simulink library "aplib"  (Simulink 10.0)
settings: Solver=VariableStepAuto  StartTime=0.0  StopTime=10.0  RelTol=1e-3
undefined symbols (not defined in the file): Aail, Aelv, Arud, Bail, Belv, Brud, Cail, CD, Celv, Crud, Dail, Delv, Drud, gamgs, HRW, Sgs, Sloc, uaero0, uprop0, xdot0, xgs, xinco, xloc, ymod1A, ymod1S, ymod2A, ymod2S, yrefA, yrefS
libraries: fdctools x42, navlib1 x8, navlib2 x2, wndlib1 x1, wndlib2 x1
(part 1 of 2)
settings Model: Creator=bhisma  LastModifiedBy=bhisma

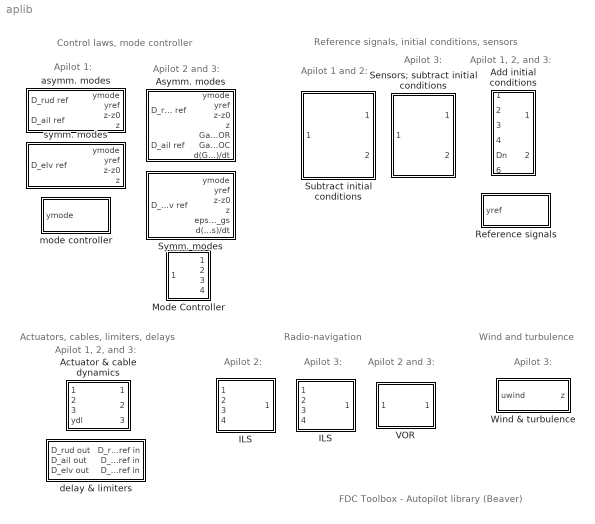
== system aplib ==
  note: Control laws, mode controller
  note: Apilot 1:
  note: Apilot 2 and 3:
  note: Reference signals, initial conditions, sensors
  note: Apilot 1, 2, and 3:
  note: Apilot 1 and 2:
  note: Apilot 3:
  note: Apilot 1, 2, and 3:
  note: Apilot 2:
  note: Radio-navigation
  note: Apilot 2 and 3:
  note: Apilot 3:
  note: FDC Toolbox - Autopilot library (Beaver)
  note: Actuators, cables, limiters, delays
  note: Apilot 3:
  note: Wind and turbulence
  Actuator & cable dynamics : Subsystem  mask(Actuator and cable dynamics){}
      mask help: Dynamics of the actuator/cable system of the Beaver autopilot system.
      mask Help: eval('browse actuatr');
      mask Display: disp('Actuator &\ncable dy-\nnamics')
  Add initial conditions : Subsystem
      mask Display: disp('Add\ninitial\ninputs')
  Asymm. modes : Subsystem  mask(Asymmetrical autopilot modes){}
      mask help:
      | Roll Attitude Hold (RAH) + turn-coordinator
      | Heading Hold/Heading Select (HH)
      | VOR navigation (NAV)
      | Localizer (LOC)
      mask Help: eval('browse ap_asymm')
      mask Display: disp('Asymmetrical\nautopilot\nmodes')
  ILS : Subsystem
      mask Display: plot(0,0,100,100,[53,23,30,61,53],[45,60,64,49,45],[16,27,32,26],[48,40,43,47],[21,20,24,26,21],[44,55,56,47,44],[20,20,16],[50,50,48],[38,27,26,33],[52,46,48,55],[42,38,27],[50,47,46],[40,44,44,45,45,44,42],[48,44,42,42,44,44,50],[47,45,43],[55,58,58],[54,84,98,90,54],[36,21,56,58,36],[74,68],[34,29],[81,76],[43,38],[87,83],[49,45],[94,89],[57,52],[105,105],[0,0])
  "ILS " : Subsystem
      mask Display: plot(0,0,100,100,[53,23,30,61,53],[45,60,64,49,45],[16,27,32,26],[48,40,43,47],[21,20,24,26,21],[44,55,56,47,44],[20,20,16],[50,50,48],[38,27,26,33],[52,46,48,55],[42,38,27],[50,47,46],[40,44,44,45,45,44,42],[48,44,42,42,44,44,50],[47,45,43],[55,58,58],[54,84,98,90,54],[36,21,56,58,36],[74,68],[34,29],[81,76],[43,38],[87,83],[49,45],[94,89],[57,52],[105,105],[0,0])
  Mode Controller : Subsystem  mask(Mode Controller){}
      mask help: Mode Controller, allows VOR navigation, Localizer, and Glideslope modes to switch from 'Armed' to 'Coupled'.
      mask Help: eval('browse modectrl')
      mask Display: disp('Mode\nCon-\ntroller')
  Reference signals : Subsystem  mask(Reference signals){}
      mask help: Reference signals for Beaver autopilot
      mask Help: eval('browse refsgnls.htm')
      mask Display: disp('Reference\nsignals')
  Sensors; subtract initial conditions : Subsystem
      mask Display: disp('Sensors\n\nsubtract\ninitial\nconditions')
  Subtract initial conditions : Subsystem
      mask Display: disp('Subtract\ninitial con-\nditions\n\nNo sensors!')
  Symm. modes : Subsystem  mask(Symmetrical autopilot modes){}
      mask help:
      | Pitch Attitude Hold (PAH) + turn-compensator
      | Altitude Hold (ALH)
      | Altitude Select (ALS)
      | Glideslope (GS)
      mask Help: eval('browse ap_symm')
      mask Display: disp('Symmetrical\nautopilot\nmodes')
  VOR : Subsystem
      mask Display: plot(0,0,100,100,[86,85,90,86,80,85,0],[16,80,20,16,20,80,62],[22,18,25,28,22,19],[36,32,29,33,36,45],[17,15,12,18,16,19],[37,37,34,32,44,46],[22,31,47,52,19,15,28,22],[36,44,39,44,55,50,45,38],[31,28],[44,45],[20,18,17],[31,30,32],[36,35,36,37,36,35,35,35,33,31,25],[41,38,33,32,30,30,32,33,37,35,34],[85,42],[80,50],[86,87,87,86,84,83,84,85],[83,81,78,76,76,79,82,83])
  Wind & turbulence : Subsystem
      mask Display: disp('Wind &\nturbulence')
  asymm. modes : Subsystem  mask(Asymmetrical autopilot modes){}
      mask help:
      | Roll Attitude Hold (RAH) + turn-coordinator
      | Heading Hold/Heading Select (HH)
      mask Help: eval('browse ap_asymm')
      mask Display: disp('Asymmetrical\nautopilot modes')
  delay & limiters : Subsystem  mask(Computational delay and limiters){}
      mask help: Computational delay and hardware-related limiters for the Beaver autopilot system.
      mask Help: eval('browse delaylim')
      mask Display: disp('Computational\ndelay & limiters')
  mode controller : Subsystem  mask(Mode Controller){}
      mask help: 'Dummy' Mode Controller (no mode-switching).
      mask Help: eval('browse modectrl')
      mask Display: disp('Mode\nController')
  symm. modes : Subsystem  mask(Symmetrical autopilot modes){}
      mask help:
      | Pitch Attitude Hold (PAH) + turn-compensator
      | Altitude Hold (ALH)
      | Altitude Select (ALS)
      mask Help: eval('browse ap_symm')
      mask Display: disp('Symmetrical\nautopilot modes')

== system aplib/Actuator & cable dynamics ==
  VDdeltae : Inport
  VDdeltaa : Inport  Port=2
  VDdeltar : Inport  Port=3
  ydl : Inport  Port=4
  Ailerons actuator and cables : StateSpace  A=Aail  B=Bail  C=Cail  D=Dail  InitialCondition=0
  Demux1 : Demux  Outputs=3
  Elevator actuator and cables : StateSpace  A=Aelv  B=Belv  C=Celv  D=Delv  InitialCondition=0
  Mux : Mux  Inputs=2
  Mux4 : Mux  Inputs=2
  Mux5 : Mux  Inputs=2
  Rudder actuator and cables : StateSpace  A=Arud  B=Brud  C=Crud  D=Drud  InitialCondition=0
  t1 : Subsystem
      settings: OpenFcn=browse actuatr
      mask Display: disp('Dynamics of the actuators and cables\nfor elevator, ailerons, and rudder.\nM.O. Rauw, January 2004')
  Ddeltae : Outport
  Ddeltaa : Outport  Port=2
  Ddeltar : Outport  Port=3
  wires:
  VDdeltae/1 -> Mux5/1
  VDdeltaa/1 -> Mux/1
  VDdeltar/1 -> Mux4/1
  Ailerons actuator and cables/1 -> Ddeltaa/1
  Rudder actuator and cables/1 -> Ddeltar/1
  Elevator actuator and cables/1 -> Ddeltae/1
  ydl/1 -> Demux1/1
  Demux1/3 -> Mux4/2  "rb/2V"
  Demux1/1 -> Mux/2  "pb/2V"
  Demux1/2 -> Mux5/2  "qc/V"
  Mux/1 -> Ailerons actuator and cables/1
  Mux4/1 -> Rudder actuator and cables/1
  Mux5/1 -> Elevator actuator and cables/1

== system aplib/Add initial conditions ==
  note: Add initial inputs
  note: ENGINE INPUTS:
  note: AERODYNAMIC INPUTS:
  Ddeltae : Inport
  Ddeltaa : Inport  Port=2
  Ddeltar : Inport  Port=3
  Ddeltaf : Inport  Port=4
  Dn : Inport  Port=5
  Dpz : Inport  Port=6
  Initial inputs for aeromod : Constant  Value=uaero0
  Initial inputs for engmod : Constant  Value=uprop0
  Mux1 : Mux
  Mux2 : Mux  Inputs=2
  Sum : Sum  SaturateOnIntegerOverflow=on  InputSameDT=on  OutDataTypeStr=Inherit: Same as first input
  Sum1 : Sum  SaturateOnIntegerOverflow=on  InputSameDT=on  OutDataTypeStr=Inherit: Same as first input
  uaero : Outport
  uprop : Outport  Port=2
  wires:
  Ddeltaa/1 -> Mux1/2
  Ddeltae/1 -> Mux1/1
  Ddeltar/1 -> Mux1/3
  Ddeltaf/1 -> Mux1/4
  Initial inputs for engmod/1 -> Sum/2
  Mux2/1 -> Sum/1
  Dpz/1 -> Mux2/2
  Dn/1 -> Mux2/1
  Initial inputs for aeromod/1 -> Sum1/1
  Sum1/1 -> uaero/1
  Mux1/1 -> Sum1/2
  Sum/1 -> uprop/1

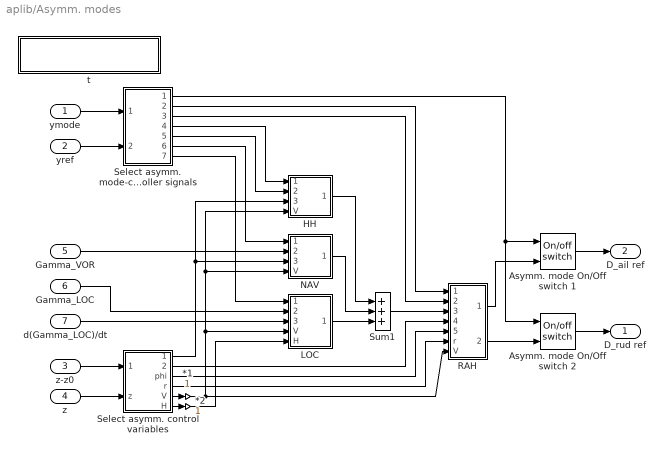
== system aplib/Asymm. modes ==
  ymode : Inport
  yref : Inport  Port=2
  z-z0 : Inport  Port=3
  z : Inport  Port=4
  Gamma_VOR : Inport  Port=5
  Gamma_LOC : Inport  Port=6
  d(Gamma_LOC)/dt : Inport  Port=7
  *1 : Gain  SaturateOnIntegerOverflow=on  OutDataTypeStr=Inherit: Same as input  ParamDataTypeStr=Inherit: Same as input
  *2 : Gain  SaturateOnIntegerOverflow=on  OutDataTypeStr=Inherit: Same as input  ParamDataTypeStr=Inherit: Same as input
  "Asymm. mode On/Off switch 1 " : fdctools/On//off switch
  Asymm. mode On/Off switch 2 : fdctools/On//off switch
  HH : Subsystem
  LOC : Subsystem
  NAV : Subsystem
  RAH : Subsystem
  Select asymm. control variables : Subsystem
  Select asymm. mode-controller signals : Subsystem
  Sum1 : Sum  Inputs=+++  SaturateOnIntegerOverflow=on  InputSameDT=on  OutDataTypeStr=Inherit: Same as first input
  t : Subsystem
      settings: OpenFcn=browse ap_asymm
      mask Display: disp('Asymm. autopilot modes\nMarc Rauw, March 2004')
  D_rud ref : Outport
  D_ail ref : Outport  Port=2
  wires:
  d(Gamma_LOC)/dt/1 -> LOC/3(d(Gamma_loc)/dt)
  Gamma_LOC/1 -> LOC/2(Gamma_loc)
  Gamma_VOR/1 -> NAV/2(Gamma_VOR)
  Select asymm. mode-controller signals/5(Dpsir (HH)) -> HH/2(Dpsir (HH))
  Sum1/1 -> RAH/3(Dphir (outer loop))
  *2/1 -> LOC/5(H)
  *1/1 -> RAH/7(V), LOC/4(V), HH/4(V), NAV/4(V)
  Select asymm. control variables/6(H) -> *2/1
  Select asymm. mode-controller signals/7(LOC coupled?) -> LOC/1(LOC coupled?)
  Select asymm. mode-controller signals/6(NAV?) -> NAV/1(NAV?)
  Select asymm. mode-controller signals/4(HH?) -> HH/1(HH?)
  Select asymm. mode-controller signals/3(Dphir (RAH)) -> RAH/2(Dphir (RAH))
  Select asymm. mode-controller signals/2(Asymm. outer loop?) -> RAH/1(Asymm.  outer loop?)
  Select asymm. control variables/2(phi-phi0) -> RAH/4(phi-phi0)
  Select asymm. control variables/3(phi) -> RAH/5(phi)
  Select asymm. control variables/4(r) -> RAH/6(r)
  Select asymm. control variables/5(V) -> *1/1
  LOC/1(Dphir (LOC)) -> Sum1/3
  NAV/1(Dphir (NAV)) -> Sum1/2
  Select asymm. control variables/1(psi-psi0) -> HH/3(psi-psi0), NAV/3(psi-psi0)
  RAH/1(D_ail ref) -> "Asymm. mode On/Off switch 1 "/2
  RAH/2(D_rud ref) -> Asymm. mode On/Off switch 2/2
  HH/1(Dphir (HH)) -> Sum1/1
  Select asymm. mode-controller signals/1(Asymm. mode?) -> "Asymm. mode On/Off switch 1 "/1, Asymm. mode On/Off switch 2/1
  ymode/1 -> Select asymm. mode-controller signals/1(ymode)
  yref/1 -> Select asymm. mode-controller signals/2(yref)
  Asymm. mode On/Off switch 2/1 -> D_rud ref/1
  "Asymm. mode On/Off switch 1 "/1 -> D_ail ref/1
  z/1 -> Select asymm. control variables/2(z)
  z-z0/1 -> Select asymm. control variables/1(z-z0)

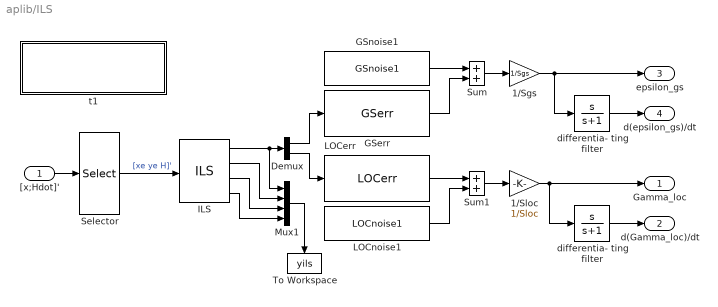
== system aplib/ILS ==
  "[x;Hdot]'" : Inport
  1/Sgs : Gain  Gain=1/Sgs  SaturateOnIntegerOverflow=on  OutDataTypeStr=Inherit: Same as input  ParamDataTypeStr=Inherit: Same as input
  1/Sloc : Gain  Gain=1/Sloc  SaturateOnIntegerOverflow=on  OutDataTypeStr=Inherit: Same as input  ParamDataTypeStr=Inherit: Same as input
  Demux : Demux  Outputs=2
  GSerr : navlib1/GSerr  cat=2  MaskParam2=0  MaskParam3=0  MaskParam4=-3
  GSnoise1 : navlib1/GSnoise1  Lgs=85  sigma_gs=15  V=30
  ILS : navlib1/ILS  RWpos=[12000,0,0]  MaskParam1=0  MaskParam3=3000  MaskParam4=300  MaskParam5=-100  MaskParam6=-3
  LOCerr : navlib1/LOCerr  cat=2  xloc=3000  MaskParam2=0  MaskParam3=0
  LOCnoise1 : navlib1/LOCnoise1  Lloc=130  sigma_loc=15  V=30
  Mux1 : Mux  Inputs=[2 2 6 2]
  Selector : Selector  InputPortWidth=13  IndexOptions=Index vector (dialog)  Indices=[10 11 12]  OutputSizes=1
  Sum : Sum  SaturateOnIntegerOverflow=on  InputSameDT=on  OutDataTypeStr=Inherit: Same as first input
  Sum1 : Sum  SaturateOnIntegerOverflow=on  InputSameDT=on  OutDataTypeStr=Inherit: Same as first input
  To Workspace : ToWorkspace  VariableName=yils
      settings: MaxDataPoints=5000
  differentia- ting filter : TransferFcn  Numerator=[1 0]  Denominator=[1 1]
  "differentia- ting filter " : TransferFcn  Numerator=[1 0]  Denominator=[1 1]
  t1 : Subsystem
      settings: OpenFcn=browse ilsxmpl
      mask Display: disp('ILS signals for autopilot\n(with noise!)\nMarc Rauw, April 2004')
  Gamma_loc : Outport
  d(Gamma_loc)/dt : Outport  Port=2
  epsilon_gs : Outport  Port=3
  d(epsilon_gs)/dt : Outport  Port=4
  wires:
  Selector/1 -> ILS/1  "[xe ye H]'"
  Demux/2 -> LOCerr/1
  Demux/1 -> GSerr/1
  Mux1/1 -> To Workspace/1
  GSnoise1/1 -> Sum/1
  GSerr/1 -> Sum/2
  Sum/1 -> 1/Sgs/1
  1/Sgs/1 -> epsilon_gs/1, differentia- ting filter/1
  differentia- ting filter/1 -> d(epsilon_gs)/dt/1
  LOCerr/1 -> Sum1/1
  LOCnoise1/1 -> Sum1/2
  1/Sloc/1 -> Gamma_loc/1, "differentia- ting filter "/1
  "differentia- ting filter "/1 -> d(Gamma_loc)/dt/1
  Sum1/1 -> 1/Sloc/1
  ILS/2 -> Mux1/2
  ILS/3 -> Mux1/3
  ILS/1 -> Mux1/1, Demux/1
  ILS/4 -> Mux1/4
  "[x;Hdot]'"/1 -> Selector/1

== system aplib/ILS  ==
  "[x;Hdot]'" : Inport
  1/Sgs : Gain  Gain=1/Sgs  SaturateOnIntegerOverflow=on  OutDataTypeStr=Inherit: Same as input  ParamDataTypeStr=Inherit: Same as input
  1/Sloc : Gain  Gain=1/Sloc  SaturateOnIntegerOverflow=on  OutDataTypeStr=Inherit: Same as input  ParamDataTypeStr=Inherit: Same as input
  Demux : Demux  Outputs=2
  GSerr : navlib1/GSerr  cat=2  MaskParam2=0  MaskParam3=0  MaskParam4=-3
  ILS : navlib1/ILS  RWpos=[12000,0,0]  MaskParam1=0  MaskParam3=3000  MaskParam4=300  MaskParam5=-100  MaskParam6=-3
  LOCerr : navlib1/LOCerr  cat=2  xloc=3000  MaskParam2=0  MaskParam3=0
  Mux1 : Mux  Inputs=[2 2 6 2]
  Selector : Selector  InputPortWidth=13  IndexOptions=Index vector (dialog)  Indices=[10 11 12]  OutputSizes=1
  To Workspace : ToWorkspace  VariableName=yils
      settings: MaxDataPoints=5000
  differentia- ting filter : TransferFcn  Numerator=[1 0]  Denominator=[1 1]
  "differentia- ting filter " : TransferFcn  Numerator=[1 0]  Denominator=[1 1]
  t1 : Subsystem
      settings: OpenFcn=browse ilsxmpl
      mask Display: disp('ILS signals for autopilot\n(no noise!)\nMarc Rauw, May 2004')
  Gamma_loc : Outport
  d(Gamma_loc)/dt : Outport  Port=2
  epsilon_gs : Outport  Port=3
  d(epsilon_gs)/dt : Outport  Port=4
  wires:
  "[x;Hdot]'"/1 -> Selector/1
  Selector/1 -> ILS/1  "[xe ye H]'"
  Mux1/1 -> To Workspace/1
  Demux/1 -> GSerr/1
  Demux/2 -> LOCerr/1
  ILS/4 -> Mux1/4
  ILS/1 -> Demux/1, Mux1/1
  ILS/3 -> Mux1/3
  ILS/2 -> Mux1/2
  GSerr/1 -> 1/Sgs/1
  1/Sgs/1 -> epsilon_gs/1, differentia- ting filter/1
  LOCerr/1 -> 1/Sloc/1
  1/Sloc/1 -> Gamma_loc/1, "differentia- ting filter "/1
  "differentia- ting filter "/1 -> d(Gamma_loc)/dt/1
  differentia- ting filter/1 -> d(epsilon_gs)/dt/1

== system aplib/Mode Controller ==
  Gamma_VOR : Inport
  d(Gamma_loc)/dt : Inport  Port=2
  Gamma_loc : Inport  Port=3
  epsilon_gs : Inport  Port=4
  Asymmetrical mode switch : Subsystem
      mask Display: disp('Armed->Coupled\nswitch for\nasymmetrical mode(s)')
  Asymmetrical mode switch1 : Subsystem
      mask Display: disp('Armed->Coupled\nswitch for\nsymmetrical mode(s)')
  GS mode active? : Constant  Value=ymod2S(5)
  GS mode status : Subsystem
      mask Display: disp('Glideslope\nmode status')
  LOC mode active? : Constant  Value=ymod2A(5)
  LOC mode status : Subsystem
      mask Display: disp('Localizer\nmode status')
  Mux1 : Mux  Inputs=[5 5]
  NAV mode active? : Constant  Value=ymod2A(4)
  NAV mode status : Subsystem
      mask Display: disp('VOR-navigation\nmode status')
  Sum : Sum  SaturateOnIntegerOverflow=on  InputSameDT=on  OutDataTypeStr=Inherit: Same as first input
  t : Subsystem
      settings: OpenFcn=browse modectrl
      mask Display: disp('Mode-controller\nM.O. Rauw, April 2004')
  ymode : Outport
  wires:
  Mux1/1 -> ymode/1
  Asymmetrical mode switch/1(ymode_asymm) -> Mux1/2
  Asymmetrical mode switch1/1(ymode_symm) -> Mux1/1
  GS mode status/1(GS status) -> Asymmetrical mode switch1/1(Symmetrical mode-status)
  epsilon_gs/1 -> GS mode status/1(epsilon_gs)
  GS mode active?/1 -> GS mode status/Enable
  Sum/1 -> Asymmetrical mode switch/1(Asymmetrical mode status)
  LOC mode status/1(LOC status) -> Sum/2
  Gamma_VOR/1 -> NAV mode status/1(Gamma_VOR)
  NAV mode active?/1 -> NAV mode status/Enable
  d(Gamma_loc)/dt/1 -> LOC mode status/2(d(Gamma_loc)/dt)
  Gamma_loc/1 -> LOC mode status/1(Gamma_loc)
  LOC mode active?/1 -> LOC mode status/Enable
  NAV mode status/1(NAV status) -> Sum/1

== system aplib/Reference signals ==
  Constant : Constant  Value=[yrefS;yrefA]
  t : Subsystem
      settings: OpenFcn=browse modectrl
      mask Display: disp('Reference signals\nMarc Rauw, April 2004')
  yref : Outport
  wires:
  Constant/1 -> yref/1

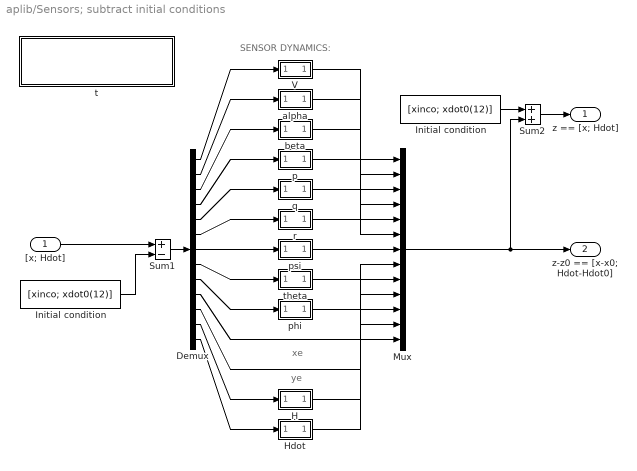
== system aplib/Sensors; subtract initial conditions ==
  note: SENSOR DYNAMICS:
  note: xe
  note: ye
  "[x; Hdot]" : Inport
  Demux : Demux  Outputs=13
  H : Subsystem
  Hdot : Subsystem
  Initial condition : Constant  Value=[xinco; xdot0(12)]
  "Initial condition " : Constant  Value=[xinco; xdot0(12)]
  Mux : Mux  Inputs=13
  Sum1 : Sum  Inputs=+-  SaturateOnIntegerOverflow=on  InputSameDT=on  OutDataTypeStr=Inherit: Same as first input
  Sum2 : Sum  SaturateOnIntegerOverflow=on  InputSameDT=on  OutDataTypeStr=Inherit: Same as first input
  V : Subsystem
  alpha : Subsystem
  beta : Subsystem
  p : Subsystem
  phi : Subsystem
  psi : Subsystem
  q : Subsystem
  r : Subsystem
  t : Subsystem
      settings: OpenFcn=browse sensors
      mask Display: disp('Include sensormodels\nhere (no VOR/ILS)!\nMarc Rauw, February 2004')
  theta : Subsystem
  "z == [x; Hdot] " : Outport
  z-z0 == [x-x0; Hdot-Hdot0] : Outport  Port=2
  wires:
  Sum1/1 -> Demux/1
  "[x; Hdot]"/1 -> Sum1/1
  Initial condition/1 -> Sum1/2
  Hdot/1(Hdot out) -> Mux/13
  H/1(H out) -> Mux/12
  V/1(V out) -> Mux/1
  alpha/1(alpha out) -> Mux/2
  beta/1(beta out) -> Mux/3
  p/1(p out) -> Mux/4
  q/1(q out) -> Mux/5
  r/1(r out) -> Mux/6
  psi/1(psi out) -> Mux/7
  theta/1(theta out) -> Mux/8
  phi/1(phi out) -> Mux/9
  Demux/13 -> Hdot/1(Hdot in)
  Demux/12 -> H/1(H in)
  Demux/11 -> Mux/11
  Demux/10 -> Mux/10
  Demux/9 -> phi/1(phi in)
  Demux/8 -> theta/1(theta in)
  Demux/7 -> psi/1(psi in)
  Demux/6 -> r/1(r in)
  Demux/5 -> q/1(q in)
  Demux/4 -> p/1(p in)
  Demux/3 -> beta/1(beta in)
  Demux/2 -> alpha/1(alpha in)
  Demux/1 -> V/1(V in)
  "Initial condition "/1 -> Sum2/1
  Sum2/1 -> "z == [x; Hdot] "/1
  Mux/1 -> Sum2/2, z-z0 == [x-x0; Hdot-Hdot0]/1

== system aplib/Subtract initial conditions ==
  note: Subtract initial conditions
  "[x; Hdot]" : Inport
  Initial condition : Constant  Value=[xinco; xdot0(12)]
  Sum : Sum  Inputs=+-  SaturateOnIntegerOverflow=on  InputSameDT=on  OutDataTypeStr=Inherit: Same as first input
  "z == [x; Hdot] " : Outport
  z-z0 == [x-x0; Hdot-Hdot0] : Outport  Port=2
  wires:
  "[x; Hdot]"/1 -> "z == [x; Hdot] "/1, Sum/1
  Initial condition/1 -> Sum/2
  Sum/1 -> z-z0 == [x-x0; Hdot-Hdot0]/1

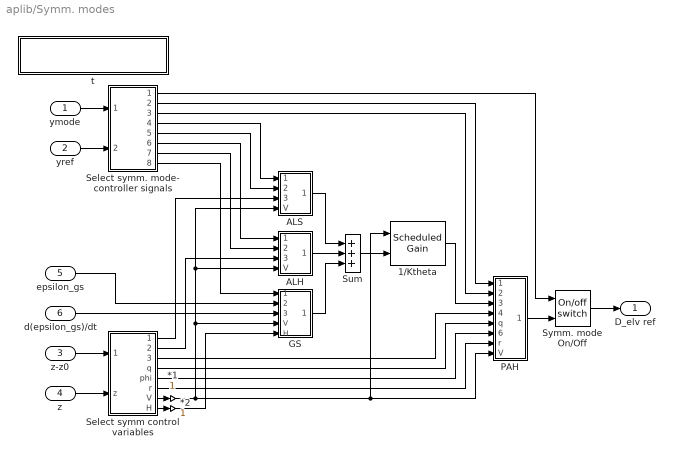
== system aplib/Symm. modes ==
  ymode : Inport
  yref : Inport  Port=2
  z-z0 : Inport  Port=3
  z : Inport  Port=4
  epsilon_gs : Inport  Port=5
  d(epsilon_gs)/dt : Inport  Port=6
  *1 : Gain  SaturateOnIntegerOverflow=on  OutDataTypeStr=Inherit: Same as input  ParamDataTypeStr=Inherit: Same as input
  *2 : Gain  SaturateOnIntegerOverflow=on  OutDataTypeStr=Inherit: Same as input  ParamDataTypeStr=Inherit: Same as input
  1/Ktheta : fdctools/Scheduled Gain  K=1/(-1.375*10^(-3)*u[1]^2 + 0.1575*u[1] - 4.8031)
  ALH : Subsystem
  ALS : Subsystem
  GS : Subsystem
  PAH : Subsystem
  Select symm control variables : Subsystem
  Select symm. mode- controller signals : Subsystem
  Sum : Sum  Inputs=+++  SaturateOnIntegerOverflow=on  InputSameDT=on  OutDataTypeStr=Inherit: Same as first input
  Symm. mode On/Off : fdctools/On//off switch
  t : Subsystem
      settings: OpenFcn=browse ap_symm
      mask Display: disp('Symm. autopilot modes\nMarc Rauw, March 2004')
  D_elv ref : Outport
  wires:
  epsilon_gs/1 -> GS/2(epsilon_gs)
  d(epsilon_gs)/dt/1 -> GS/3(d(epsilon_gs)/dt)
  *1/1 -> ALS/4(V), ALH/4(V), GS/4(V), PAH/8(V), 1/Ktheta/1
  1/Ktheta/1 -> PAH/3(Dthetar (outer loop))
  GS/1(Dthetar (GS)) -> Sum/3
  ALS/1(Dthetar (ALS)) -> Sum/1
  ALH/1(Dthetar (ALH)) -> Sum/2
  Select symm control variables/1(Hdot-Hdot0) -> ALS/3(Hdot-Hdot0)
  Select symm control variables/2(H-H0) -> ALH/3(H-H0)
  Select symm control variables/3(theta-theta0) -> PAH/4(theta-theta0)
  Select symm control variables/4(q) -> PAH/5(q)
  Select symm control variables/5(phi) -> PAH/6(phi)
  Select symm control variables/6(r) -> PAH/7(r)
  Select symm control variables/7(V) -> *1/1
  Select symm. mode- controller signals/2(Symm. outer loop?) -> PAH/1(Symm.  outer loop?)
  Select symm. mode- controller signals/3(Dthetar (PAH)) -> PAH/2(Dthetar (PAH/GA))
  Select symm. mode- controller signals/4(ALS?) -> ALS/1(ALS?)
  Select symm. mode- controller signals/5(DHdot r (ALS)) -> ALS/2(DHdot r (ALS))
  Select symm. mode- controller signals/6(ALH?) -> ALH/1(ALH?)
  Select symm. mode- controller signals/7(DHr (ALH)) -> ALH/2(DHr (ALH))
  Select symm control variables/8(H) -> *2/1
  *2/1 -> GS/5(H)
  Select symm. mode- controller signals/8(GS coupled?) -> GS/1(GS coupled?)
  Select symm. mode- controller signals/1(Symm. mode?) -> Symm. mode On/Off/1
  PAH/1(D_elv ref) -> Symm. mode On/Off/2
  Symm. mode On/Off/1 -> D_elv ref/1
  yref/1 -> Select symm. mode- controller signals/2(yref)
  ymode/1 -> Select symm. mode- controller signals/1(ymode)
  z-z0/1 -> Select symm control variables/1(z-z0)
  z/1 -> Select symm control variables/2(z)
  Sum/1 -> 1/Ktheta/2

== system aplib/VOR ==
  "[x' ; Hdot]'" : Inport
  Demux : Demux  Outputs=[3 1]
  Mux1 : Mux  Inputs=[1 1 2 1]
  Selector : Selector  InputPortWidth=13  IndexOptions=Index vector (dialog)  Indices=[10 11 12 7]  OutputSizes=1
  To Workspace : ToWorkspace  VariableName=yvor
      settings: MaxDataPoints=5000
  VOR : navlib2/VOR  xVOR=xVOR  yVOR=yVOR  HVOR=HVOR  CD=CD
  VORerr : navlib2/VORerr  MaskParam1=0
  t : Subsystem
      settings: OpenFcn=browse vorxmpl
      mask Display: disp('VOR signals\nMarc Rauw, February 2004')
  Gamma_VOR : Outport
  wires:
  "[x' ; Hdot]'"/1 -> Selector/1
  Selector/1 -> Demux/1
  Demux/1 -> VOR/1  "[xe ye H]'"
  Demux/2 -> VOR/2  "psi"
  VORerr/1 -> Mux1/1, Gamma_VOR/1
  VOR/4 -> Mux1/4
  VOR/3 -> Mux1/3
  VOR/2 -> Mux1/2
  Mux1/1 -> To Workspace/1
  VOR/1 -> VORerr/1

== system aplib/Wind & turbulence ==
  z : Inport
  BLwind : wndlib1/BLwind  Vw=1*(u[1]^0.2545 - 0.4097)/1.3470  psi_w=180  theta_w=0
  Demux : Demux  Outputs=[12 1]
  Demux1 : Demux  Outputs=[1 11]
  Mux1 : Mux  Inputs=[3 3]
  Sum : Sum  SaturateOnIntegerOverflow=on  InputSameDT=on  OutDataTypeStr=Inherit: Same as first input
  Terminator_1 : Terminator
  Terminator_2 : Terminator
  deriv : Derivative
  t : Subsystem
      mask Display: disp('Wind and turbulence\nMarc Rauw, April 2003')
  turb2 : wndlib2/turb2
  uwind : Outport
  wires:
  BLwind/1 -> deriv/1, Mux1/1
  deriv/1 -> Mux1/2
  Sum/1 -> uwind/1
  turb2/1 -> Sum/1
  Mux1/1 -> Sum/2
  Demux1/1 -> turb2/1  "V"
  Demux1/2 -> Terminator_2/1
  z/1 -> Demux/1
  Demux/1 -> Demux1/1, BLwind/1  "x"
  Demux/2 -> Terminator_1/1

== system aplib/asymm. modes ==
  ymode : Inport
  yref : Inport  Port=2
  z-z0 : Inport  Port=3
  z : Inport  Port=4
  *1 : Gain  SaturateOnIntegerOverflow=on  OutDataTypeStr=Inherit: Same as input  ParamDataTypeStr=Inherit: Same as input
  "Asymm. mode On/Off switch 1 " : fdctools/On//off switch
  Asymm. mode On/Off switch 2 : fdctools/On//off switch
  HH : Subsystem
  RAH : Subsystem
  Select asymm. control variables : Subsystem
  Select asymm. mode-controller signals : Subsystem
  Terminator_1 : Terminator
  Terminator_2 : Terminator
  Terminator_3 : Terminator
  t : Subsystem
      settings: OpenFcn=browse ap_asymm
      mask Display: disp('Asymm. autopilot modes\n(without NAV and LOC modes)\nMarc Rauw, April 2003')
  D_rud ref : Outport
  D_ail ref : Outport  Port=2
  wires:
  *1/1 -> RAH/7(V), HH/4(V)
  RAH/2(D_rud ref) -> Asymm. mode On/Off switch 2/2
  Select asymm. control variables/5(V) -> *1/1
  Select asymm. control variables/4(r) -> RAH/6(r)
  z/1 -> Select asymm. control variables/2(z)
  HH/1(Dphir (HH)) -> RAH/3(Dphir (outer loop))
  Select asymm. control variables/1(psi-psi0) -> HH/3(psi-psi0)
  RAH/1(D_ail ref) -> "Asymm. mode On/Off switch 1 "/2
  Select asymm. control variables/6(H) -> Terminator_1/1
  Asymm. mode On/Off switch 2/1 -> D_rud ref/1
  "Asymm. mode On/Off switch 1 "/1 -> D_ail ref/1
  z-z0/1 -> Select asymm. control variables/1(z-z0)
  Select asymm. control variables/2(phi-phi0) -> RAH/4(phi-phi0)
  Select asymm. control variables/3(phi) -> RAH/5(phi)
  Select asymm. mode-controller signals/2(Asymm. outer loop?) -> RAH/1(Asymm.  outer loop?)
  yref/1 -> Select asymm. mode-controller signals/2(yref)
  ymode/1 -> Select asymm. mode-controller signals/1(ymode)
  Select asymm. mode-controller signals/1(Asymm. mode?) -> Asymm. mode On/Off switch 2/1, "Asymm. mode On/Off switch 1 "/1
  Select asymm. mode-controller signals/3(Dphir (RAH)) -> RAH/2(Dphir (RAH))
  Select asymm. mode-controller signals/4(HH?) -> HH/1(HH?)
  Select asymm. mode-controller signals/5(Dpsir (HH)) -> HH/2(Dpsir (HH))
  Select asymm. mode-controller signals/6(NAV?) -> Terminator_2/1
  Select asymm. mode-controller signals/7(LOC coupled?) -> Terminator_3/1

== system aplib/delay & limiters ==
  D_rud ref in : Inport
  D_ail ref in : Inport  Port=2
  D_elv ref in : Inport  Port=3
  " +/- 10 V " : Saturate  UpperLimit=10 * (pi/180)  LowerLimit=-10 * (pi/180)
  " delay" : TransportDelay  DelayTime=0.03
  +/- 10 V : Saturate  UpperLimit=10 * (pi/180)  LowerLimit=-10 * (pi/180)
  "+/- 10 V " : Saturate  UpperLimit=10 * (pi/180)  LowerLimit=-10 * (pi/180)
  delay : TransportDelay  DelayTime=0.03
  "delay " : TransportDelay  DelayTime=0.03
  t : Subsystem
      settings: OpenFcn=browse delaylim
      mask Display: disp('Computational delay and\ninput limiters (+- 10 Volt)\nMarc Rauw, April 2003')
  D_rud out : Outport
  D_ail out : Outport  Port=2
  D_elv out : Outport  Port=3
  wires:
  D_rud ref in/1 -> delay/1
  delay/1 -> +/- 10 V/1
  D_elv ref in/1 -> " delay"/1
  " +/- 10 V "/1 -> D_elv out/1
  D_ail ref in/1 -> "delay "/1
  "+/- 10 V "/1 -> D_ail out/1
  +/- 10 V/1 -> D_rud out/1
  " delay"/1 -> " +/- 10 V "/1
  "delay "/1 -> "+/- 10 V "/1

== system aplib/mode controller ==
  Mux1 : Mux  Inputs=[5 5]
  asymm. mode-switches : Constant  Value=ymod1A
  symm. mode-switches : Constant  Value=ymod1S
  t : Subsystem
      settings: OpenFcn=browse modectrl
      mask Display: disp('Mode Controller (Mode Select)\nNo on-line mode-switching!\nMarc Rauw, April 2003')
  ymode : Outport
  wires:
  Mux1/1 -> ymode/1
  symm. mode-switches/1 -> Mux1/1
  asymm. mode-switches/1 -> Mux1/2

== system aplib/symm. modes ==
  ymode : Inport
  yref : Inport  Port=2
  z-z0 : Inport  Port=3
  z : Inport  Port=4
  *1 : Gain  SaturateOnIntegerOverflow=on  OutDataTypeStr=Inherit: Same as input  ParamDataTypeStr=Inherit: Same as input
  1/Ktheta : fdctools/Scheduled Gain  K=1/(-1.375*10^(-3)*u[1]^2 + 0.1575*u[1] - 4.8031)
  ALH : Subsystem
  ALS : Subsystem
  PAH : Subsystem
  Select symm control variables : Subsystem
  Select symm. mode- controller signals : Subsystem
  Sum : Sum  SaturateOnIntegerOverflow=on  InputSameDT=on  OutDataTypeStr=Inherit: Same as first input
  Symm. mode On/Off : fdctools/On//off switch
  Terminator_1 : Terminator
  Terminator_2 : Terminator
  t : Subsystem
      settings: OpenFcn=browse ap_symm
      mask Display: disp('Symm. autopilot modes\n(without glideslope mode)\nMarc Rauw, April 2003')
  D_elv ref : Outport
  wires:
  Symm. mode On/Off/1 -> D_elv ref/1
  PAH/1(D_elv ref) -> Symm. mode On/Off/2
  ALH/1(Dthetar (ALH)) -> Sum/2
  Select symm control variables/2(H-H0) -> ALH/3(H-H0)
  Select symm control variables/3(theta-theta0) -> PAH/4(theta-theta0)
  Select symm control variables/4(q) -> PAH/5(q)
  Select symm control variables/5(phi) -> PAH/6(phi)
  Select symm control variables/6(r) -> PAH/7(r)
  Select symm control variables/7(V) -> *1/1
  Select symm. mode- controller signals/4(ALS?) -> ALS/1(ALS?)
  Select symm. mode- controller signals/5(DHdot r (ALS)) -> ALS/2(DHdot r (ALS))
  Select symm. mode- controller signals/6(ALH?) -> ALH/1(ALH?)
  Select symm. mode- controller signals/7(DHr (ALH)) -> ALH/2(DHr (ALH))
  Select symm. mode- controller signals/3(Dthetar (PAH)) -> PAH/2(Dthetar (PAH/GA))
  Select symm. mode- controller signals/2(Symm. outer loop?) -> PAH/1(Symm.  outer loop?)
  Select symm. mode- controller signals/1(Symm. mode?) -> Symm. mode On/Off/1
  Select symm control variables/1(Hdot-Hdot0) -> ALS/3(Hdot-Hdot0)
  *1/1 -> ALS/4(V), ALH/4(V), PAH/8(V), 1/Ktheta/1
  ALS/1(Dthetar (ALS)) -> Sum/1
  1/Ktheta/1 -> PAH/3(Dthetar (outer loop))
  Select symm control variables/8(H) -> Terminator_1/1
  Select symm. mode- controller signals/8(GS coupled?) -> Terminator_2/1
  yref/1 -> Select symm. mode- controller signals/2(yref)
  ymode/1 -> Select symm. mode- controller signals/1(ymode)
  z-z0/1 -> Select symm control variables/1(z-z0)
  z/1 -> Select symm control variables/2(z)
  Sum/1 -> 1/Ktheta/2

== system aplib/Actuator & cable dynamics/t1 ==

== system aplib/Asymm. modes/HH ==
  note: Heading Hold / Heading Select mode
  HH? : Inport
  Dpsir (HH) : Inport  Port=2
  psi-psi0 : Inport  Port=3
  V : Inport  Port=4
  Kpsi : fdctools/Scheduled Gain  K=0.05*u[1] - 1.1
  On/Off : fdctools/On//off switch
  Sum : Sum  Inputs=+-  SaturateOnIntegerOverflow=on  InputSameDT=on  OutDataTypeStr=Inherit: Same as first input
  Dphir (HH) : Outport
  wires:
  V/1 -> Kpsi/1
  HH?/1 -> On/Off/1
  Dpsir (HH)/1 -> Sum/1
  psi-psi0/1 -> Sum/2
  Kpsi/1 -> On/Off/2
  Sum/1 -> Kpsi/2
  On/Off/1 -> Dphir (HH)/1

== system aplib/Asymm. modes/LOC ==
  note: Localizer coupled mode
  LOC coupled? : Inport
  Gamma_loc : Inport  Port=2
  d(Gamma_loc)/dt : Inport  Port=3
  V : Inport  Port=4
  H : Inport  Port=5
  KGam_LOC : fdctools/Scheduled Gain  K=(7.75*10^(-3)*u[1]^2 - 0.76*u[1] + 15.75625)/1000
  Kv : Gain  Gain=10  SaturateOnIntegerOverflow=on  OutDataTypeStr=Inherit: Same as input  ParamDataTypeStr=Inherit: Same as input
  On/Off : fdctools/On//off switch
  Rloc approximation : Fcn  Expr=(u[1]-HRW)/sin(abs(gamgs*pi/180)) + xloc - xgs
  Sum : Sum  SaturateOnIntegerOverflow=on  InputSameDT=on  OutDataTypeStr=Inherit: Same as first input
  prod : Product  SaturateOnIntegerOverflow=on  RndMeth=Zero  InputSameDT=on  OutDataTypeStr=Inherit: Same as first input
  Dphir (LOC) : Outport
  wires:
  V/1 -> KGam_LOC/1
  Gamma_loc/1 -> Sum/1
  Kv/1 -> Sum/2
  d(Gamma_loc)/dt/1 -> Kv/1
  Sum/1 -> prod/1
  H/1 -> Rloc approximation/1
  prod/1 -> KGam_LOC/2
  KGam_LOC/1 -> On/Off/2
  LOC coupled?/1 -> On/Off/1
  On/Off/1 -> Dphir (LOC)/1
  Rloc approximation/1 -> prod/2

== system aplib/Asymm. modes/NAV ==
  note: VOR navigation mode
  NAV? : Inport
  Gamma_VOR : Inport  Port=2
  psi-psi0 : Inport  Port=3
  V : Inport  Port=4
  Dpsir (NAV) : Constant  Value=CD-xinco(7)
  KGam_VOR : fdctools/Scheduled Gain  K=5.375*10^(-2)*u[1]^2 - 6.825*u[1] + 153.03125
  Kpsi : fdctools/Scheduled Gain  K=0.05*u[1] - 1.1
  Low-pass filter : TransferFcn  Denominator=[1 1]
  On/Off : fdctools/On//off switch
  Sum : Sum  SaturateOnIntegerOverflow=on  InputSameDT=on  OutDataTypeStr=Inherit: Same as first input
  Sum1 : Sum  Inputs=+-  SaturateOnIntegerOverflow=on  InputSameDT=on  OutDataTypeStr=Inherit: Same as first input
  Washout filter : TransferFcn  Numerator=[15 0]  Denominator=[15 1]
  Dphir (NAV) : Outport
  wires:
  V/1 -> Kpsi/1, KGam_VOR/1
  psi-psi0/1 -> Sum1/2
  NAV?/1 -> On/Off/1
  Sum/1 -> On/Off/2
  Washout filter/1 -> Sum/2
  Kpsi/1 -> Washout filter/1
  Low-pass filter/1 -> Sum/1
  KGam_VOR/1 -> Low-pass filter/1
  Gamma_VOR/1 -> KGam_VOR/2
  Sum1/1 -> Kpsi/2
  Dpsir (NAV)/1 -> Sum1/1
  On/Off/1 -> Dphir (NAV)/1

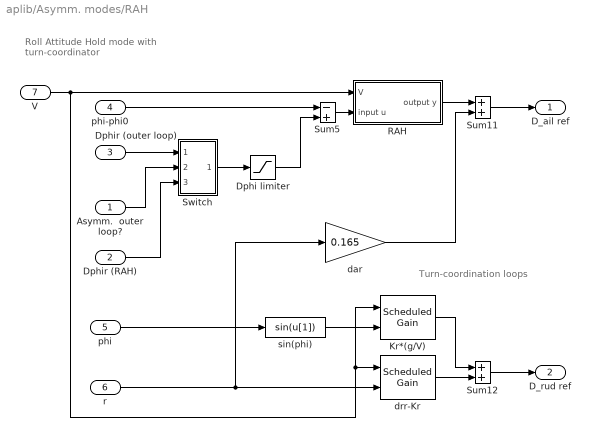
== system aplib/Asymm. modes/RAH ==
  note: Turn-coordination loops
  note: Roll Attitude Hold mode
      | with turn-coordinator
  Asymm.  outer loop? : Inport
  Dphir (RAH) : Inport  Port=2
  Dphir (outer loop) : Inport  Port=3
  phi-phi0 : Inport  Port=4
  phi : Inport  Port=5
  r : Inport  Port=6
  V : Inport  Port=7
  Dphi limiter : Saturate  UpperLimit=30*pi/180  LowerLimit=-30*pi/180
  Kr*(g/V) : fdctools/Scheduled Gain  K=-4*(9.80665/u[1])
  RAH : Subsystem
      mask Display: disp('RAH (limited \n PI controller)')
  Sum11 : Sum  SaturateOnIntegerOverflow=on  InputSameDT=on  OutDataTypeStr=Inherit: Same as first input
  Sum12 : Sum  SaturateOnIntegerOverflow=on  InputSameDT=on  OutDataTypeStr=Inherit: Same as first input
  Sum5 : Sum  Inputs=-+  SaturateOnIntegerOverflow=on  InputSameDT=on  OutDataTypeStr=Inherit: Same as first input
  Switch : Subsystem
      mask Display: plot(0,0,100,100,[100,70,40,0],[50,50,80,80],[40,0],[20,20],[29,29,0],[64,50,50],[29,29],[36,50],[40,40,41,40,39,40],[80,82,80,78,80,82],[40,40,41,40,39,40],[19,21,20,18,20,23])
  dar : Gain  Gain=0.165  SaturateOnIntegerOverflow=on  OutDataTypeStr=Inherit: Same as input  ParamDataTypeStr=Inherit: Same as input
  drr-Kr : fdctools/Scheduled Gain  K=(-7.5*10^(-5)*u[1]^2 + 0.0095*u[1] - 0.4606) + 4
  sin(phi) : Fcn
  D_ail ref : Outport
  D_rud ref : Outport  Port=2
  wires:
  V/1 -> RAH/1(V), Kr*(g/V)/1, drr-Kr/1
  phi-phi0/1 -> Sum5/1
  Switch/1(Dphir) -> Dphi limiter/1
  RAH/1(output y) -> Sum11/1
  Sum11/1 -> D_ail ref/1
  dar/1 -> Sum11/2
  Sum5/1 -> RAH/2(input u)
  Dphi limiter/1 -> Sum5/2
  Dphir (outer loop)/1 -> Switch/1(Dphir (outer loop))
  Asymm.  outer loop?/1 -> Switch/2(Asymm.  outer loop?)
  Dphir (RAH)/1 -> Switch/3(Dphir (RAH))
  phi/1 -> sin(phi)/1
  Sum12/1 -> D_rud ref/1
  drr-Kr/1 -> Sum12/2
  Kr*(g/V)/1 -> Sum12/1
  sin(phi)/1 -> Kr*(g/V)/2
  r/1 -> dar/1, drr-Kr/2

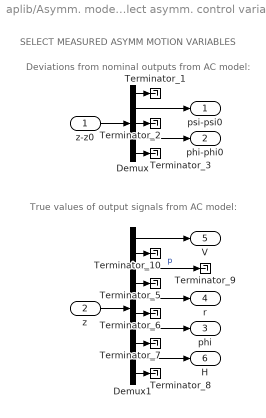
== system aplib/Asymm. modes/Select asymm. control variables ==
  note: SELECT MEASURED ASYMM MOTION VARIABLES
  note: Deviations from nominal outputs from AC model:
  note: True values of output signals from AC model:
  z-z0 : Inport
  z : Inport  Port=2
  Demux : Demux  Outputs=[6 1 1 1 4]
  Demux1 : Demux  Outputs=[1 2 1 1 1 2 1 2 1 1]
  Terminator_{1..3,5..10} (9 alike) : Terminator
  psi-psi0 : Outport
  phi-phi0 : Outport  Port=2
  phi : Outport  Port=3
  r : Outport  Port=4
  V : Outport  Port=5
  H : Outport  Port=6
  wires:
  Demux/5 -> Terminator_3/1
  z-z0/1 -> Demux/1
  Demux/2 -> psi-psi0/1
  Demux/4 -> phi-phi0/1
  Demux/1 -> Terminator_1/1
  Demux/3 -> Terminator_2/1
  Demux1/9 -> H/1
  z/1 -> Demux1/1
  Demux1/3 -> Terminator_9/1  "p"
  Demux1/5 -> r/1
  Demux1/7 -> phi/1
  Demux1/2 -> Terminator_10/1
  Demux1/4 -> Terminator_5/1
  Demux1/6 -> Terminator_6/1
  Demux1/8 -> Terminator_7/1
  Demux1/10 -> Terminator_8/1
  Demux1/1 -> V/1

== system aplib/Asymm. modes/Select asymm. mode-controller signals ==
  note: SELECT ASYMM MODE
      | (on/off flags denoted by '?')
  note: SELECT ASYMM REFERENCE SIGNALS
  ymode : Inport
  yref : Inport  Port=2
  Demux : Demux  Outputs=[5 1 1 1 1 1]
  Demux1 : Demux  Outputs=[3 1 1]
  Terminator_1 : Terminator
  Terminator_2 : Terminator
  Asymm. mode? : Outport
  Asymm. outer loop? : Outport  Port=2
  Dphir (RAH) : Outport  Port=3
  HH? : Outport  Port=4
  Dpsir (HH) : Outport  Port=5
  NAV? : Outport  Port=6
  LOC coupled? : Outport  Port=7
  wires:
  ymode/1 -> Demux/1
  Demux/2 -> Asymm. mode?/1
  Demux/3 -> Asymm. outer loop?/1
  Demux/4 -> HH?/1
  Demux/5 -> NAV?/1
  Demux/6 -> LOC coupled?/1
  Demux/1 -> Terminator_1/1
  yref/1 -> Demux1/1
  Demux1/2 -> Dphir (RAH)/1
  Demux1/3 -> Dpsir (HH)/1
  Demux1/1 -> Terminator_2/1

== system aplib/Asymm. modes/t ==

== system aplib/ILS/t1 ==

== system aplib/ILS /t1 ==

== system aplib/Mode Controller/Asymmetrical mode switch ==
  note: Switch from 'armed'/initial mode to 'coupled'/final mode when
      | mode-status changes from positive value to negative value. If no
      | 'switchable' asymmetrical mode is selected, the mode-status will
      | be equal to zero, and only the 'initial' mode will be active.
  note: Armed -> Coupled switch for asymmetrical mode(s)
  Asymmetrical mode status : Inport
  Mux5 : Mux  Inputs=5
  "Switch " : Switch  SaturateOnIntegerOverflow=on  InputSameDT=on
  asymm mode-setting ('armed'/initial mode) : Constant  Value=ymod1A
  asymm mode-setting ('coupled'/final mode) : Constant  Value=ymod2A
  ymode_asymm : Outport
  wires:
  "Switch "/1 -> ymode_asymm/1
  Mux5/1 -> "Switch "/2
  asymm mode-setting ('armed'/initial mode)/1 -> "Switch "/1
  asymm mode-setting ('coupled'/final mode)/1 -> "Switch "/3
  Asymmetrical mode status/1 -> Mux5/2, Mux5/1, Mux5/4, Mux5/5, Mux5/3

== system aplib/Mode Controller/Asymmetrical mode switch1 ==
  note: Switch from 'armed'/initial mode to 'coupled'/final mode when
      | mode-status changes from positive value to negative value. If no
      | 'switchable' asymmetrical mode is selected, the mode-status will
      | be equal to zero, and only the 'initial' mode will be active.
  note: Armed -> Coupled switch for symmetrical mode(s)
  Symmetrical mode-status : Inport
  Mux4 : Mux  Inputs=5
  Switch : Switch  SaturateOnIntegerOverflow=on  InputSameDT=on
  symm mode-setting ('armed'/initial mode) : Constant  Value=ymod1S
  symm mode-setting ('coupled'/final mode) : Constant  Value=ymod2S
  ymode_symm : Outport
  wires:
  Mux4/1 -> Switch/2
  symm mode-setting ('armed'/initial mode)/1 -> Switch/1
  symm mode-setting ('coupled'/final mode)/1 -> Switch/3
  Symmetrical mode-status/1 -> Mux4/4, Mux4/5, Mux4/2, Mux4/1, Mux4/3
  Switch/1 -> ymode_symm/1

== system aplib/Mode Controller/GS mode status ==
  note: Determine Glideslope mode status (armed or coupled)
  note: GS status equals 1 if GS is armed,
      | and equals -1 if GS is coupled.
  epsilon_gs : Inport
  Enable : EnablePort
  Memory : Memory  InitialCondition=1
  Mux2 : Mux  Inputs=2
  gsswitch.m : MATLABFcn  MATLABFcn=gsswitch  OutputDimensions=1  OutputSignalType=real
  GS status : Outport
  wires:
  gsswitch.m/1 -> Memory/1, GS status/1
  Mux2/1 -> gsswitch.m/1
  Memory/1 -> Mux2/2
  epsilon_gs/1 -> Mux2/1

== system aplib/Mode Controller/LOC mode status ==
  note: Determine Localizer mode status (armed or coupled)
  note: LOC status equals 1 if LOC is armed,
      | and equals -1 if LOC is coupled.
  Gamma_loc : Inport
  d(Gamma_loc)/dt : Inport  Port=2
  Enable : EnablePort
  " Memory" : Memory  InheritSampleTime=on
  Mux : Mux  Inputs=3
  locswtch.m : MATLABFcn  MATLABFcn=locswtch  OutputDimensions=1
  LOC status : Outport
  wires:
  locswtch.m/1 -> " Memory"/1, LOC status/1
  " Memory"/1 -> Mux/3
  d(Gamma_loc)/dt/1 -> Mux/2
  Gamma_loc/1 -> Mux/1
  Mux/1 -> locswtch.m/1

== system aplib/Mode Controller/NAV mode status ==
  note: Determine VOR-navigation mode status (armed or coupled)
  note: NAV status equals 1 if NAV is armed,
      | and equals -1 if NAV is coupled.
  Gamma_VOR : Inport
  Enable : EnablePort
  "Memory " : Memory  InitialCondition=1  InheritSampleTime=on
  Mux2 : Mux  Inputs=2
  navswtch.m : MATLABFcn  MATLABFcn=navswtch  OutputDimensions=1
  NAV status : Outport
  wires:
  Mux2/1 -> navswtch.m/1
  navswtch.m/1 -> NAV status/1, "Memory "/1
  "Memory "/1 -> Mux2/2
  Gamma_VOR/1 -> Mux2/1

== system aplib/Mode Controller/t ==

== system aplib/Reference signals/t ==

== system aplib/Sensors; subtract initial conditions/H ==
  note: Transport delay in static system,
      | selection between continuous
      | altitude signal, quantized signal
      | (Least significant bit of 4 feet),
      | and quantized, but averaged signal
  H in : Inport
  1 = cont. signal 2 = 4ft quantizer 3 = MA-filter : Constant
  4ft quantizer : Subsystem  mask(Quantizer){q=4*0.3048}
      mask prompts: q "Quantization interval:"
      mask help: Discretizes input at given interval.
      mask Help: Quantizes input in given intervals.
      mask Display: plot([10,0],[5,5],[5,5],[0,10],[1,2,2,3,3,4,4,5,5,6,6,7,7,8,8,9,9],[1,1,2,2,3,3,4,4,5,5,6,6,7,7,8,8,9])
  MA-filter : fdctools/MA-filter  ns=10  Ts=0.033  uinit=0
  Multiport Switch : MultiPortSwitch  SaturateOnIntegerOverflow=on  InputSameDT=on
  Transport delay static pressure : TransportDelay  DelayTime=0.4
  H out : Outport
  wires:
  4ft quantizer/1(Out1) -> MA-filter/1, Multiport Switch/3
  MA-filter/1 -> Multiport Switch/4
  1 = cont. signal 2 = 4ft quantizer 3 = MA-filter/1 -> Multiport Switch/1
  Transport delay static pressure/1 -> Multiport Switch/2, 4ft quantizer/1(In1)
  Multiport Switch/1 -> H out/1
  H in/1 -> Transport delay static pressure/1

== system aplib/Sensors; subtract initial conditions/Hdot ==
  Hdot in : Inport
  Pressure delay/ computing time airdata computer : TransportDelay  DelayTime=0.8
  Hdot out : Outport
  wires:
  Hdot in/1 -> Pressure delay/ computing time airdata computer/1
  Pressure delay/ computing time airdata computer/1 -> Hdot out/1

== system aplib/Sensors; subtract initial conditions/V ==
  V in : Inport
  Transport Delay pitot system : TransportDelay  DelayTime=0.4
  V out : Outport
  wires:
  V in/1 -> Transport Delay pitot system/1
  Transport Delay pitot system/1 -> V out/1

== system aplib/Sensors; subtract initial conditions/alpha ==
  alpha in : Inport
  alpha out : Outport
  wires:
  alpha in/1 -> alpha out/1

== system aplib/Sensors; subtract initial conditions/beta ==
  beta in : Inport
  beta out : Outport
  wires:
  beta in/1 -> beta out/1

== system aplib/Sensors; subtract initial conditions/p ==
  p in : Inport
  p out : Outport
  wires:
  p in/1 -> p out/1

== system aplib/Sensors; subtract initial conditions/phi ==
  phi in : Inport
  phi out : Outport
  wires:
  phi in/1 -> phi out/1

== system aplib/Sensors; subtract initial conditions/psi ==
  psi in : Inport
  psi out : Outport
  wires:
  psi in/1 -> psi out/1

== system aplib/Sensors; subtract initial conditions/q ==
  q in : Inport
  q out : Outport
  wires:
  q in/1 -> q out/1

== system aplib/Sensors; subtract initial conditions/r ==
  r in : Inport
  r out : Outport
  wires:
  r in/1 -> r out/1

== system aplib/Sensors; subtract initial conditions/t ==

== system aplib/Sensors; subtract initial conditions/theta ==
  theta in : Inport
  theta out : Outport
  wires:
  theta in/1 -> theta out/1

== system aplib/Symm. modes/ALH ==
  note: Altitude Hold mode
  ALH? : Inport
  DHr (ALH) : Inport  Port=2
  H-H0 : Inport  Port=3
  V : Inport  Port=4
  KH : fdctools/Scheduled Gain  K=(-1.0*10^(-4)*u[1]^2 + 0.015*u[1] - 0.5975)*(pi/180)
  On/Off : fdctools/On//off switch
  Sum : Sum  Inputs=+-  SaturateOnIntegerOverflow=on  InputSameDT=on  OutDataTypeStr=Inherit: Same as first input
  Dthetar (ALH) : Outport
  wires:
  V/1 -> KH/1
  Sum/1 -> KH/2
  KH/1 -> On/Off/2
  ALH?/1 -> On/Off/1
  DHr (ALH)/1 -> Sum/1
  On/Off/1 -> Dthetar (ALH)/1
  H-H0/1 -> Sum/2

== system aplib/Symm. modes/ALS ==
  note: Altitude Select Mode
  ALS? : Inport
  DHdot r (ALS) : Inport  Port=2
  Hdot-Hdot0 : Inport  Port=3
  V : Inport  Port=4
  KHdot : fdctools/Scheduled Gain  K=(-3.875*10^(-4)*u[1]^2 + 0.04025*u[1] - 1.1041)*(pi/180)
  On/Off : fdctools/On//off switch
  Sum : Sum  Inputs=+-  SaturateOnIntegerOverflow=on  InputSameDT=on  OutDataTypeStr=Inherit: Same as first input
  filter : TransferFcn  Denominator=[1 0.15]
  Dthetar (ALS) : Outport
  wires:
  V/1 -> KHdot/1
  Hdot-Hdot0/1 -> Sum/2
  KHdot/1 -> On/Off/2
  ALS?/1 -> On/Off/1
  DHdot r (ALS)/1 -> Sum/1
  On/Off/1 -> Dthetar (ALS)/1
  Sum/1 -> filter/1
  filter/1 -> KHdot/2

== system aplib/Symm. modes/GS ==
  note: Glideslope coupled mode
  GS coupled? : Inport
  epsilon_gs : Inport  Port=2
  d(epsilon_gs)/dt : Inport  Port=3
  V : Inport  Port=4
  H : Inport  Port=5
  Keps_gs : fdctools/Scheduled Gain  K=(0.00575*u[1]^2 - 0.63*u[1] + 18.00625)/1000
  Kr : Gain  SaturateOnIntegerOverflow=on  OutDataTypeStr=Inherit: Same as input  ParamDataTypeStr=Inherit: Same as input
  On/Off : fdctools/On//off switch
  Rgs approximation : Fcn  Expr=(u[1]-HRW)/sin(abs(gamgs*pi/180))
  Sum : Sum  SaturateOnIntegerOverflow=on  InputSameDT=on  OutDataTypeStr=Inherit: Same as first input
  prod : Product  SaturateOnIntegerOverflow=on  RndMeth=Zero  InputSameDT=on  OutDataTypeStr=Inherit: Same as first input
  Dthetar (GS) : Outport
  wires:
  On/Off/1 -> Dthetar (GS)/1
  Keps_gs/1 -> On/Off/2
  prod/1 -> Keps_gs/2
  Rgs approximation/1 -> prod/2
  Sum/1 -> prod/1
  Kr/1 -> Sum/2
  d(epsilon_gs)/dt/1 -> Kr/1
  epsilon_gs/1 -> Sum/1
  V/1 -> Keps_gs/1
  GS coupled?/1 -> On/Off/1
  H/1 -> Rgs approximation/1

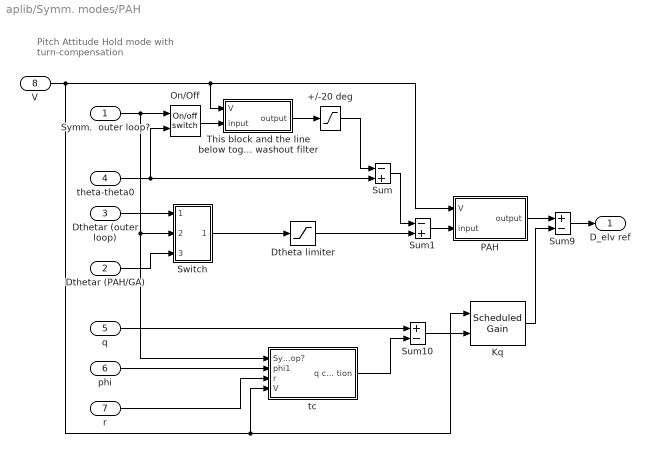
== system aplib/Symm. modes/PAH ==
  note: Pitch Attitude Hold mode
      | with turn-compensation
  Symm.  outer loop? : Inport
  Dthetar (PAH/GA) : Inport  Port=2
  Dthetar (outer loop) : Inport  Port=3
  theta-theta0 : Inport  Port=4
  q : Inport  Port=5
  phi : Inport  Port=6
  r : Inport  Port=7
  V : Inport  Port=8
  +/-20 deg : Saturate  UpperLimit=20*(pi/180)  LowerLimit=-20*(pi/180)
  Dtheta limiter : Saturate  UpperLimit=18*(pi/180)  LowerLimit=-8*(pi/180)
  Kq : fdctools/Scheduled Gain  K=-4.75*10^(-4)*u[1]^2 +0.0540*u[1] - 1.5931
  On/Off : fdctools/On//off switch
  PAH : Subsystem
      mask Display: disp('PAH (limited \n PI controller)')
  Sum : Sum  Inputs=-+  SaturateOnIntegerOverflow=on  InputSameDT=on  OutDataTypeStr=Inherit: Same as first input
  Sum1 : Sum  Inputs=-+  SaturateOnIntegerOverflow=on  InputSameDT=on  OutDataTypeStr=Inherit: Same as first input
  Sum10 : Sum  Inputs=+-  SaturateOnIntegerOverflow=on  InputSameDT=on  OutDataTypeStr=Inherit: Same as first input
  Sum9 : Sum  Inputs=+-  SaturateOnIntegerOverflow=on  InputSameDT=on  OutDataTypeStr=Inherit: Same as first input
  Switch : Subsystem
      mask Display: plot(0,0,100,100,[100,70,40,0],[50,50,80,80],[40,0],[20,20],[29,29,0],[64,50,50],[29,29],[36,50],[40,40,41,40,39,40],[80,82,80,78,80,82],[40,40,41,40,39,40],[19,21,20,18,20,23])
  This block and the line below together form a washout filter : Subsystem
      mask Display: disp('Kd/(s+Kd)')
  tc : Subsystem
      mask Display: disp('Turn\nCompensator')
  D_elv ref : Outport
  wires:
  Dthetar (outer loop)/1 -> Switch/1(Dthetar (outer loop))
  Switch/1(Dthetar) -> Dtheta limiter/1
  Sum1/1 -> PAH/2(input)
  Dtheta limiter/1 -> Sum1/2
  PAH/1(output) -> Sum9/1
  Kq/1 -> Sum9/2
  Sum/1 -> Sum1/1
  +/-20 deg/1 -> Sum/1
  theta-theta0/1 -> Sum/2, On/Off/2
  Dthetar (PAH/GA)/1 -> Switch/3(Dthetar (PAH/GA))
  r/1 -> tc/3(r)
  phi/1 -> tc/2(phi1)
  Sum10/1 -> Kq/2
  q/1 -> Sum10/1
  tc/1(q correc- tion) -> Sum10/2
  Sum9/1 -> D_elv ref/1
  Symm.  outer loop?/1 -> On/Off/1, tc/1(Symm. outer loop?), Switch/2(Symm.  outer loop?)
  This block and the line below together form a washout filter/1(output) -> +/-20 deg/1
  On/Off/1 -> This block and the line below together form a washout filter/2(input)
  V/1 -> Kq/1, tc/4(V), PAH/1(V), This block and the line below together form a washout filter/1(V)

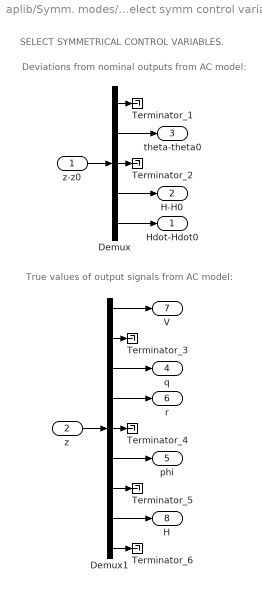
== system aplib/Symm. modes/Select symm control variables ==
  note: SELECT SYMMETRICAL CONTROL VARIABLES.
  note: True values of output signals from AC model:
  note: Deviations from nominal outputs from AC model:
  z-z0 : Inport
  z : Inport  Port=2
  Demux : Demux  Outputs=[7 1 3 1 1]
  Demux1 : Demux  Outputs=[1 3 1 1 2 1 2 1 1]
  Terminator_{1..6} (6 alike) : Terminator
  Hdot-Hdot0 : Outport
  H-H0 : Outport  Port=2
  theta-theta0 : Outport  Port=3
  q : Outport  Port=4
  phi : Outport  Port=5
  r : Outport  Port=6
  V : Outport  Port=7
  H : Outport  Port=8
  wires:
  Demux/1 -> Terminator_1/1
  z-z0/1 -> Demux/1
  Demux/3 -> Terminator_2/1
  Demux/5 -> Hdot-Hdot0/1
  Demux/4 -> H-H0/1
  Demux/2 -> theta-theta0/1
  Demux1/1 -> V/1
  z/1 -> Demux1/1
  Demux1/2 -> Terminator_3/1
  Demux1/5 -> Terminator_4/1
  Demux1/7 -> Terminator_5/1
  Demux1/9 -> Terminator_6/1
  Demux1/4 -> r/1
  Demux1/6 -> phi/1
  Demux1/8 -> H/1
  Demux1/3 -> q/1

== system aplib/Symm. modes/Select symm. mode- controller signals ==
  note: SELECT SYMMETRICAL MODE
      | (on/off flags denoted by '?')
  note: SELECT SYMM REFERENCE SIGNALS
  ymode : Inport
  yref : Inport  Port=2
  Demux : Demux  Outputs=[1 1 1 1 1 5]
  Demux1 : Demux  Outputs=[1 1 1 2]
  Terminator_1 : Terminator
  Terminator_2 : Terminator
  Symm. mode? : Outport
  Symm. outer loop? : Outport  Port=2
  Dthetar (PAH) : Outport  Port=3
  ALS? : Outport  Port=4
  DHdot r (ALS) : Outport  Port=5
  ALH? : Outport  Port=6
  DHr (ALH) : Outport  Port=7
  GS coupled? : Outport  Port=8
  wires:
  Demux1/4 -> Terminator_2/1
  Demux1/3 -> DHdot r (ALS)/1
  Demux1/2 -> DHr (ALH)/1
  Demux1/1 -> Dthetar (PAH)/1
  yref/1 -> Demux1/1
  Demux/5 -> GS coupled?/1
  Demux/4 -> ALS?/1
  Demux/3 -> ALH?/1
  Demux/1 -> Symm. mode?/1
  Demux/2 -> Symm. outer loop?/1
  ymode/1 -> Demux/1
  Demux/6 -> Terminator_1/1

== system aplib/Symm. modes/t ==

== system aplib/VOR/t ==

== system aplib/Wind & turbulence/t ==

== system aplib/asymm. modes/HH ==
  note: Heading Hold / Heading Select mode
  HH? : Inport
  Dpsir (HH) : Inport  Port=2
  psi-psi0 : Inport  Port=3
  V : Inport  Port=4
  Kpsi : fdctools/Scheduled Gain  K=0.05*u[1] - 1.1
  On/Off : fdctools/On//off switch
  Sum : Sum  Inputs=+-  SaturateOnIntegerOverflow=on  InputSameDT=on  OutDataTypeStr=Inherit: Same as first input
  Dphir (HH) : Outport
  wires:
  V/1 -> Kpsi/1
  HH?/1 -> On/Off/1
  Dpsir (HH)/1 -> Sum/1
  psi-psi0/1 -> Sum/2
  Kpsi/1 -> On/Off/2
  Sum/1 -> Kpsi/2
  On/Off/1 -> Dphir (HH)/1

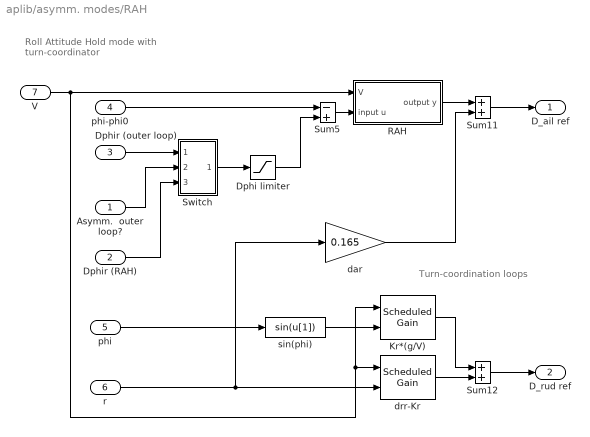
== system aplib/asymm. modes/RAH ==
  note: Turn-coordination loops
  note: Roll Attitude Hold mode
      | with turn-coordinator
  Asymm.  outer loop? : Inport
  Dphir (RAH) : Inport  Port=2
  Dphir (outer loop) : Inport  Port=3
  phi-phi0 : Inport  Port=4
  phi : Inport  Port=5
  r : Inport  Port=6
  V : Inport  Port=7
  Dphi limiter : Saturate  UpperLimit=30*pi/180  LowerLimit=-30*pi/180
  Kr*(g/V) : fdctools/Scheduled Gain  K=-4*(9.80665/u[1])
  RAH : Subsystem
      mask Display: disp('RAH (limited \n PI controller)')
  Sum11 : Sum  SaturateOnIntegerOverflow=on  InputSameDT=on  OutDataTypeStr=Inherit: Same as first input
  Sum12 : Sum  SaturateOnIntegerOverflow=on  InputSameDT=on  OutDataTypeStr=Inherit: Same as first input
  Sum5 : Sum  Inputs=-+  SaturateOnIntegerOverflow=on  InputSameDT=on  OutDataTypeStr=Inherit: Same as first input
  Switch : Subsystem
      mask Display: plot(0,0,100,100,[100,70,40,0],[50,50,80,80],[40,0],[20,20],[29,29,0],[64,50,50],[29,29],[36,50],[40,40,41,40,39,40],[80,82,80,78,80,82],[40,40,41,40,39,40],[19,21,20,18,20,23])
  dar : Gain  Gain=0.165  SaturateOnIntegerOverflow=on  OutDataTypeStr=Inherit: Same as input  ParamDataTypeStr=Inherit: Same as input
  drr-Kr : fdctools/Scheduled Gain  K=(-7.5*10^(-5)*u[1]^2 + 0.0095*u[1] - 0.4606) + 4
  sin(phi) : Fcn
  D_ail ref : Outport
  D_rud ref : Outport  Port=2
  wires:
  V/1 -> RAH/1(V), Kr*(g/V)/1, drr-Kr/1
  phi-phi0/1 -> Sum5/1
  Switch/1(Dphir) -> Dphi limiter/1
  RAH/1(output y) -> Sum11/1
  Sum11/1 -> D_ail ref/1
  dar/1 -> Sum11/2
  Sum5/1 -> RAH/2(input u)
  Dphi limiter/1 -> Sum5/2
  Dphir (outer loop)/1 -> Switch/1(Dphir (outer loop))
  Asymm.  outer loop?/1 -> Switch/2(Asymm.  outer loop?)
  Dphir (RAH)/1 -> Switch/3(Dphir (RAH))
  phi/1 -> sin(phi)/1
  Sum12/1 -> D_rud ref/1
  drr-Kr/1 -> Sum12/2
  Kr*(g/V)/1 -> Sum12/1
  sin(phi)/1 -> Kr*(g/V)/2
  r/1 -> dar/1, drr-Kr/2
